simulink model "Model_Controlled_sys"  (R2024b)
settings: Solver=VariableStepAuto  StartTime=0.0  StopTime=150  RelTol=1e-3
undefined symbols (not defined in the file or in its folder): drv
settings Model: Creator=federico  LastModifiedBy=Buton

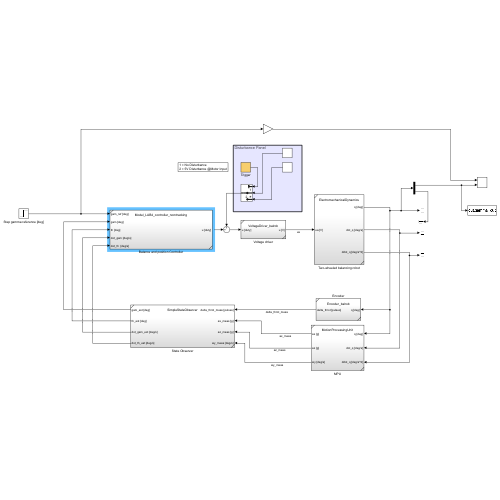
[thumbnail: Simulink's stored preview of the top-level diagram]
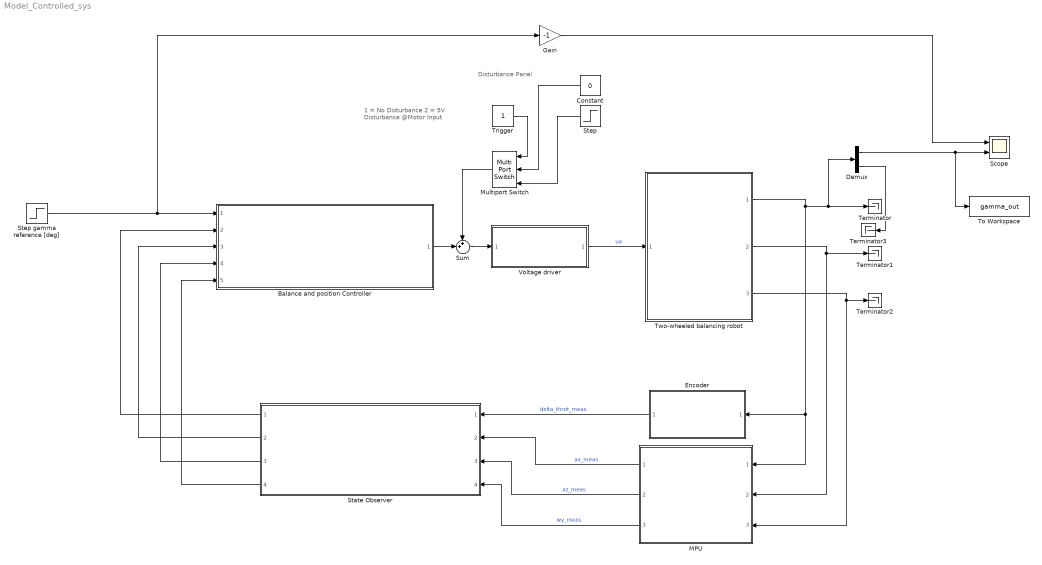
== system Model_Controlled_sys ==
  note: 1 = No Disturbance
      | 2 = 5V Disturbance @Motor Input
  note: Disturbance Panel
  Balance and position Controller : Subsystem  ReferencedSubsystem=Model_LAB4_controller_nomtracking
  Constant : Constant  Value=0
  Demux : Demux  Outputs=2
  Encoder : Subsystem  ReferencedSubsystem=Encoder_balrob
  Gain : Gain  Gain=-1
  MPU : Subsystem  ReferencedSubsystem=MotionProcessingUnit
  Multiport Switch : MultiPortSwitch  Inputs=2  SaturateOnIntegerOverflow=off  InputSameDT=off
  Scope : Scope  NumInputPorts=2
  State Observer : Subsystem  ReferencedSubsystem=SimpleStateObserver
  Step : Step  Time=10  After=5/drv.duty2V  SampleTime=0
  Step gamma reference [deg] : Step  Time=0  After=168.517  SampleTime=0
  Sum : Sum  Inputs=++|
  Terminator{,1..3} (4 alike) : Terminator
  To Workspace : ToWorkspace  VariableName=gamma_out  SaveFormat=Timeseries  SampleTime=-1
  Trigger : Constant
  Two-wheeled balancing robot : Subsystem  ReferencedSubsystem=ElectromechanicalDynamics
  Voltage driver : Subsystem  ReferencedSubsystem=VoltageDriver_balrob
  wires:
  Encoder/1 -> State Observer/1  "delta_throt_meas"
  Two-wheeled balancing robot/3 -> MPU/3, Terminator2/1
  Two-wheeled balancing robot/1 -> MPU/1, Encoder/1, Terminator/1, Demux/1
  MPU/2 -> State Observer/3  "az_meas"
  MPU/3 -> State Observer/4  "wy_meas"
  Voltage driver/1 -> Two-wheeled balancing robot/1  "ua"
  Two-wheeled balancing robot/2 -> Terminator1/1, MPU/2
  MPU/1 -> State Observer/2  "ax_meas"
  State Observer/1 -> Balance and position Controller/2
  State Observer/2 -> Balance and position Controller/3
  State Observer/3 -> Balance and position Controller/4
  State Observer/4 -> Balance and position Controller/5
  Sum/1 -> Voltage driver/1
  Balance and position Controller/1 -> Sum/2
  Multiport Switch/1 -> Sum/1
  Trigger/1 -> Multiport Switch/1
  Constant/1 -> Multiport Switch/2
  Step/1 -> Multiport Switch/3
  Step gamma reference [deg]/1 -> Gain/1, Balance and position Controller/1
  Demux/1 -> To Workspace/1, Scope/2
  Demux/2 -> Terminator3/1
  Gain/1 -> Scope/1
